simulink model "motor_model_sys_id"  (R2018a)
settings: Solver=FixedStepAuto  StartTime=0.0  StopTime=10.0  FixedStep=0.001  RelTol=1e-3
undefined symbols (not defined in the file): b, J, K, L, R
settings Model: Creator=greedyhao  LastModifiedBy=greedyhao

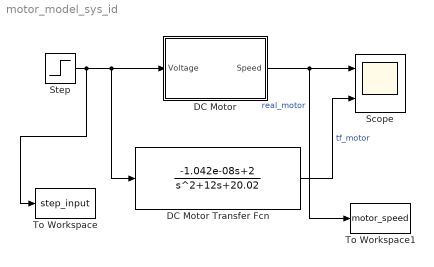
== system motor_model_sys_id ==
  DC Motor : Subsystem
  DC Motor Transfer Fcn : TransferFcn  Numerator=[-1.042e-08 2]  Denominator=[1 12 20.02]
  Scope : Scope  NumInputPorts=2
  Step : Step  Time=0.3  SampleTime=0
  To Workspace : ToWorkspace  VariableName=step_input  SampleTime=-1
      settings: Save2DSignal=2-D array (concatenate along first dimension)
  To Workspace1 : ToWorkspace  VariableName=motor_speed  SampleTime=-1
      settings: Save2DSignal=2-D array (concatenate along first dimension)
  wires:
  DC Motor/1(Speed) -> To Workspace1/1, Scope/1  "real_motor"
  Step/1 -> To Workspace/1, DC Motor Transfer Fcn/1, DC Motor/1(Voltage)
  DC Motor Transfer Fcn/1 -> Scope/2  "tf_motor"

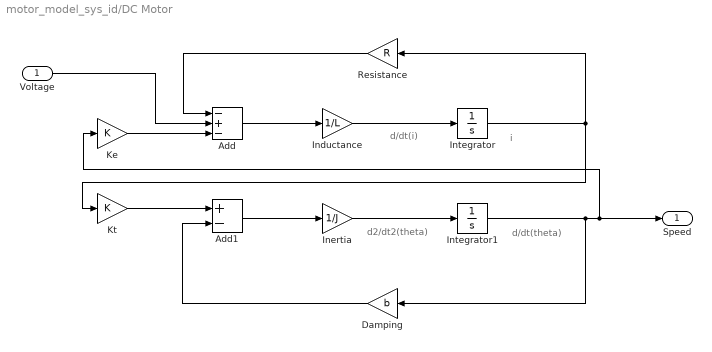
== system motor_model_sys_id/DC Motor ==
  note: i
  note: d/dt(i)
  note: d/dt(theta)
  note: d2/dt2(theta)
  Voltage : Inport
  Add : Sum  Inputs=-+-
  Add1 : Sum  Inputs=+-
  Damping : Gain  Gain=b
  Inductance : Gain  Gain=1/L
  Inertia : Gain  Gain=1/J
  Integrator : Integrator
  Integrator1 : Integrator
  Ke : Gain  Gain=K
  Kt : Gain  Gain=K
  Resistance : Gain  Gain=R
  Speed : Outport
  wires:
  Inductance/1 -> Integrator/1
  Integrator1/1 -> Damping/1, Speed/1, Ke/1
  Inertia/1 -> Integrator1/1
  Integrator/1 -> Resistance/1, Kt/1
  Kt/1 -> Add1/1
  Voltage/1 -> Add/2
  Resistance/1 -> Add/1
  Damping/1 -> Add1/2
  Ke/1 -> Add/3
  Add/1 -> Inductance/1
  Add1/1 -> Inertia/1
